simulink subsystem "ElectricalThermalSystem"  (R2024a)
settings: Solver=VariableStepAuto  StartTime=0.0  StopTime=10.0  RelTol=1e-3
undefined symbols (not defined in the file): PlantThrEstCmpPwr, PlntDCDCMass, PlntEMCp, PlntThrAirBpt, PlntThrAirCond, PlntThrAirCp, PlntThrAirCpBpt, PlntThrAirPrand, PlntThrAirRho, PlntThrAirVisc, PlntThrBattDCFlwRatio, PlntThrBattJacArea, PlntThrBattJacLen, PlntThrChArea, PlntThrChDia, PlntThrConvCoeff, PlntThrCoolCond, PlntThrCoolCp, PlntThrCoolCpBpt, PlntThrCoolPrand, PlntThrCoolRho, PlntThrCoolVisc, PlntThrDCJacArea, PlntThrDCJacLen, PlntThrEMJacArea, PlntThrEMJacLen, PlntThrEstCOPLut, PlntThrEstDTLut, PlntThrFanDisp, PlntThrFanMaxSpd, PlntThrFanMechEff, PlntThrFanNomP, PlntThrFanVolEff, PlntThrHeaterMaxPwr, PlntThrHtVsCurr, PlntThrHtVsCurrBpt, PlntThrPmpDisp, PlntThrPmpHeadP, PlntThrPmpMaxSpd, PlntThrPmpMechEff, PlntThrPmpVolEff, PlntThrRadAirArea, PlntThrRadAirDh, PlntThrRadFanAreaFlw, PlntThrRadFlwCoef, PlntThrRadGapHeight, PlntThrRadLength, PlntThrRadNTubes, PlntThrRadTubeDh, PlntThrRadTubeHeight, PlntThrRadWidth
libraries: simulink x5, autolibsharedcommon x1, autolibutils x1
settings Model: ModifiedByFormat=The MathWorks, Inc.  Creator=The MathWorks, Inc.  LastModifiedBy=The MathWorks, Inc.
settings RTWCC: GPUComputeCapability=3.5  LargeConstantGeneration=WriteOnlyDNNConstantsToDataFiles

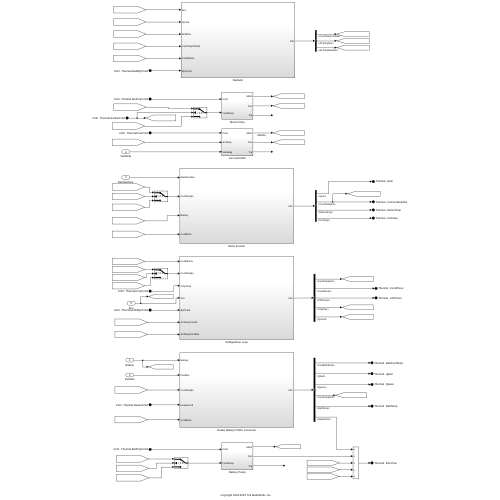
[thumbnail: Simulink's stored preview of the top-level diagram]
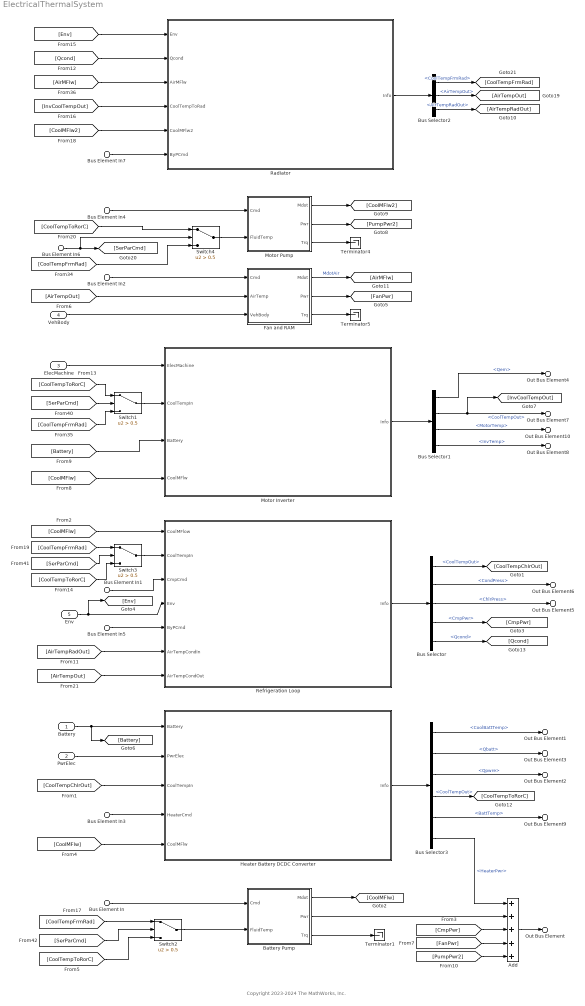
== system ElectricalThermalSystem ==
  note: Copyright 2023-2024 The MathWorks, Inc.
  Battery : Inport
  PwrElec : Inport  Port=2
  ElecMachine : Inport  Port=3
  VehBody : Inport  Port=4
  Env : Inport  Port=5
  Bus Element In : Inport  Port=6  PortName=Cntrl  Element=Thermal.BattPmpCmd
  Bus Element In1 : Inport  Port=6  PortName=Cntrl  Element=Thermal.CmpCmd
  Bus Element In2 : Inport  Port=6  PortName=Cntrl  Element=Thermal.FanCmd
  Bus Element In3 : Inport  Port=6  PortName=Cntrl  Element=Thermal.HeaterCmd
  Bus Element In4 : Inport  Port=6  PortName=Cntrl  Element=Thermal.MotPmpCmd
  Bus Element In5 : Inport  Port=6  PortName=Cntrl  Element=Thermal.ChlrByPCmd
  Bus Element In6 : Inport  Port=6  PortName=Cntrl  Element=Thermal.SerParCmd
  Bus Element In7 : Inport  Port=6  PortName=Cntrl  Element=Thermal.RadByPCmd
  Add : Sum  Inputs=+++++
  Battery Pump : Subsystem
  Bus Selector : BusSelector  OutputSignals=CoolTempOut,CondPress,ChlrPress,CmpPwr,Qcond
  Bus Selector1 : BusSelector  OutputSignals=Qem,CoolTempOut,MotorTemp,InvTemp
  Bus Selector2 : BusSelector  OutputSignals=CoolTempFrmRad,AirTempOut,AirTempRadOut
  Bus Selector3 : BusSelector  OutputSignals=CoolBattTemp,Qbatt,Qpwre,CoolTempOut,BattTemp,HeaterPwr
  Fan and RAM : Subsystem
  Heater Battery DCDC Converter : Subsystem
  Motor Inverter : Subsystem
  Motor Pump : Subsystem
  Radiator : Subsystem
  Refrigeration Loop : Subsystem
  Switch{1..4} (4 alike) : Switch  Criteria=u2 > Threshold  Threshold=0.5  SaturateOnIntegerOverflow=off  InputSameDT=off
  Terminator1 : Terminator
  Terminator4 : Terminator
  Terminator5 : Terminator
  Out Bus Element7 : Outport  PortName=Thermal  Element=InvCoolTempOut
  Out Bus Element8 : Outport  PortName=Thermal  Element=InvTemp
  Out Bus Element9 : Outport  PortName=Thermal  Element=BattTemp
  Out Bus Element10 : Outport  PortName=Thermal  Element=MotorTemp
  Out Bus Element5 : Outport  PortName=Thermal  Element=ChlrPress
  Out Bus Element6 : Outport  PortName=Thermal  Element=CondPress
  Out Bus Element : Outport  PortName=Thermal  Element=EAccPwr
  Out Bus Element1 : Outport  PortName=Thermal  Element=BattCoolTemp
  Out Bus Element3 : Outport  PortName=Thermal  Element=Qbatt
  Out Bus Element2 : Outport  PortName=Thermal  Element=Qpwre
  Out Bus Element4 : Outport  PortName=Thermal  Element=Qem
  wires:
  [CoolTempFrmRad] -> Switch4/3
  [CoolTempToRorC] -> Switch4/1
  [CoolTempToRorC] -> Switch2/3
  [CoolTempFrmRad] -> Switch2/1
  [CoolTempFrmRad] -> Switch1/3
  [CoolTempToRorC] -> Switch1/1
  [CoolTempToRorC] -> Switch3/3
  [CoolTempFrmRad] -> Switch3/1
  Bus Selector3/6 -> Add/1  "<HeaterPwr>"
  Battery Pump/2(Pwr) -> Add/2
  [CmpPwr] -> Add/3
  [FanPwr] -> Add/4
  [PumpPwr2] -> Add/5
  Bus Selector1/4 -> Out Bus Element8/1  "<InvTemp>"
  Bus Selector3/5 -> Out Bus Element9/1  "<BattTemp>"
  Bus Selector1/3 -> Out Bus Element10/1  "<MotorTemp>"
  Bus Selector/1 -> [CoolTempChlrOut]  "<CoolTempOut>"
  Bus Selector2/1 -> [CoolTempFrmRad]  "<CoolTempFrmRad>"
  [CoolMFlw2] -> Radiator/5(CoolMFlw2)
  Switch4/1 -> Motor Pump/2(FluidTemp)
  Bus Element In6/1 -> Switch4/2, [SerParCmd]
  Switch3/1 -> Refrigeration Loop/2(CoolTempIn)
  [SerParCmd] -> Switch3/2
  Switch2/1 -> Battery Pump/2(FluidTemp)
  [SerParCmd] -> Switch2/2
  [SerParCmd] -> Switch1/2
  Switch1/1 -> Motor Inverter/2(CoolTempIn)
  Bus Selector2/2 -> [AirTempOut]  "<AirTempOut>"
  Radiator/1(Info) -> Bus Selector2/1
  [InvCoolTempOut] -> Radiator/4(CoolTempToRad)
  [AirMFlw] -> Radiator/3(AirMFlw)
  [Qcond] -> Radiator/2(Qcond)
  [Env] -> Radiator/1(Env)
  Refrigeration Loop/1(Info) -> Bus Selector/1
  Bus Selector/5 -> [Qcond]  "<Qcond>"
  Motor Pump/1(Mdot) -> [CoolMFlw2]
  Motor Pump/2(Pwr) -> [PumpPwr2]
  Motor Pump/3(Trq) -> Terminator4/1
  Bus Element In4/1 -> Motor Pump/1(Cmd)
  Bus Selector1/2 -> Out Bus Element7/1, [InvCoolTempOut]  "<CoolTempOut>"
  Bus Selector1/1 -> Out Bus Element4/1  "<Qem>"
  Motor Inverter/1(Info) -> Bus Selector1/1
  [Battery] -> Motor Inverter/3(Battery)
  [CoolMFlw] -> Motor Inverter/4(CoolMFlw)
  VehBody/1 -> Fan and RAM/3(VehBody)
  Fan and RAM/3(Trq) -> Terminator5/1
  Fan and RAM/2(Pwr) -> [FanPwr]
  Fan and RAM/1(Mdot) -> [AirMFlw]  "MdotAir"
  Bus Element In2/1 -> Fan and RAM/1(Cmd)
  [AirTempOut] -> Fan and RAM/2(AirTemp)
  [CoolMFlw] -> Heater Battery DCDC Converter/5(CoolMFlw)
  Add/1 -> Out Bus Element/1
  Bus Selector/3 -> Out Bus Element5/1  "<ChlrPress>"
  Bus Selector/2 -> Out Bus Element6/1  "<CondPress>"
  Bus Selector/4 -> [CmpPwr]  "<CmpPwr>"
  [CoolTempChlrOut] -> Heater Battery DCDC Converter/3(CoolTempIn)
  Env/1 -> Refrigeration Loop/4(Env), [Env]
  Bus Element In1/1 -> Refrigeration Loop/3(CmpCmd)
  [CoolMFlw] -> Refrigeration Loop/1(CoolMFlow)
  Bus Selector3/4 -> [CoolTempToRorC]  "<CoolTempOut>"
  Bus Selector3/3 -> Out Bus Element2/1  "<Qpwre>"
  Bus Selector3/2 -> Out Bus Element3/1  "<Qbatt>"
  Bus Selector3/1 -> Out Bus Element1/1  "<CoolBattTemp>"
  Heater Battery DCDC Converter/1(Info) -> Bus Selector3/1
  Bus Element In3/1 -> Heater Battery DCDC Converter/4(HeaterCmd)
  Battery Pump/3(Trq) -> Terminator1/1
  Battery Pump/1(Mdot) -> [CoolMFlw]
  Bus Element In/1 -> Battery Pump/1(Cmd)
  ElecMachine/1 -> Motor Inverter/1(ElecMachine)
  PwrElec/1 -> Heater Battery DCDC Converter/2(PwrElec)
  Battery/1 -> [Battery], Heater Battery DCDC Converter/1(Battery)
  Bus Element In7/1 -> Radiator/6(ByPCmd)
  Bus Element In5/1 -> Refrigeration Loop/5(ByPCmd)
  Bus Selector2/3 -> [AirTempRadOut]  "<AirTempRadOut>"
  [AirTempRadOut] -> Refrigeration Loop/6(AirTempCondIn)
  [AirTempOut] -> Refrigeration Loop/7(AirTempCondOut)

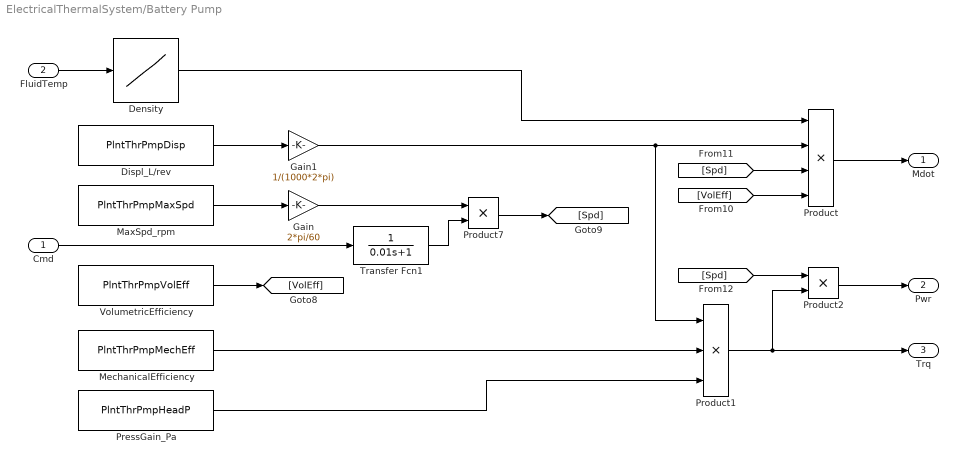
== system ElectricalThermalSystem/Battery Pump ==
  Cmd : Inport
  FluidTemp : Inport  Port=2
  Density : Lookup_n-D  NumberOfTableDimensions=1  BreakpointsForDimension1=PlntThrCoolCpBpt  Table=PlntThrCoolRho  ExtrapMethod=Clip  UseLastTableValue=on  InternalRulePriority=Speed  RndMeth=Simplest
  Displ_L/rev : Constant  Value=PlntThrPmpDisp  SampleTime=-1
  Gain : Gain  Gain=2*pi/60
  Gain1 : Gain  Gain=1/(1000*2*pi)
  MaxSpd_rpm : Constant  Value=PlntThrPmpMaxSpd  SampleTime=-1
  MechanicalEfficiency : Constant  Value=PlntThrPmpMechEff  SampleTime=-1
  PressGain_Pa : Constant  Value=PlntThrPmpHeadP  SampleTime=-1
  Product : Product  Inputs=4
  Product1 : Product  Inputs=3
  Product2 : Product
  Product7 : Product
  Transfer Fcn1 : TransferFcn  Denominator=[0.01 1]
  VolumetricEfficiency : Constant  Value=PlntThrPmpVolEff  SampleTime=-1
  Mdot : Outport
  Pwr : Outport  Port=2
  Trq : Outport  Port=3
  wires:
  Product2/1 -> Pwr/1
  Cmd/1 -> Transfer Fcn1/1
  Product/1 -> Mdot/1
  Gain1/1 -> Product/2, Product1/1
  Product1/1 -> Product2/2, Trq/1
  PressGain_Pa/1 -> Product1/3
  [Spd] -> Product2/1
  MechanicalEfficiency/1 -> Product1/2
  [VolEff] -> Product/4
  [Spd] -> Product/3
  Product7/1 -> [Spd]
  Displ_L/rev/1 -> Gain1/1
  Gain/1 -> Product7/1
  MaxSpd_rpm/1 -> Gain/1
  Density/1 -> Product/1
  VolumetricEfficiency/1 -> [VolEff]
  FluidTemp/1 -> Density/1
  Transfer Fcn1/1 -> Product7/2

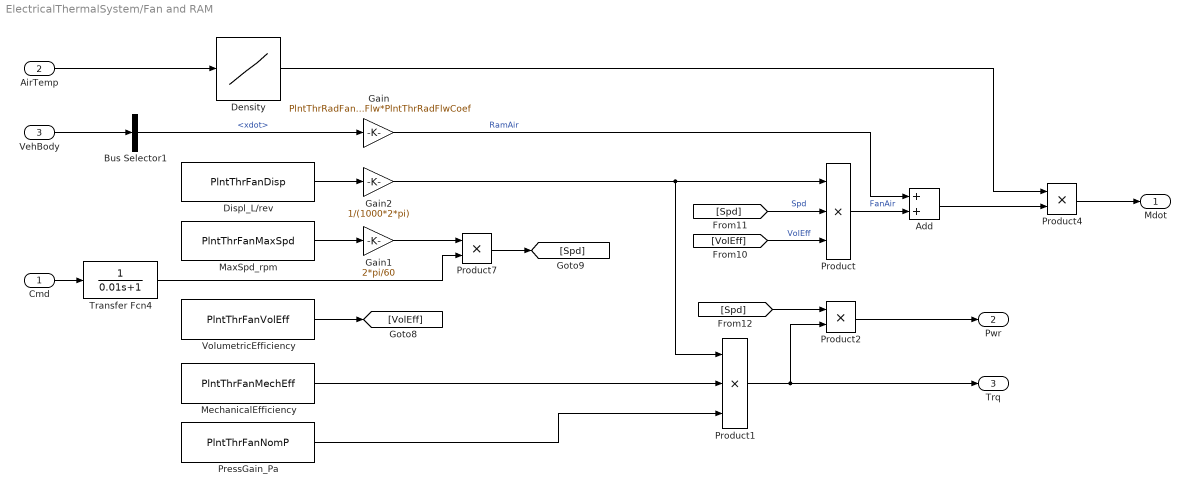
== system ElectricalThermalSystem/Fan and RAM ==
  Cmd : Inport
  AirTemp : Inport  Port=2
  VehBody : Inport  Port=3
  Add : Sum
  Bus Selector1 : BusSelector  OutputSignals=BdyFrm.Cg.Vel.xdot
  Density : Lookup_n-D  NumberOfTableDimensions=1  BreakpointsForDimension1=PlntThrAirBpt  Table=PlntThrAirRho  ExtrapMethod=Clip  UseLastTableValue=on  InternalRulePriority=Speed  RndMeth=Simplest
  Displ_L/rev : Constant  Value=PlntThrFanDisp  SampleTime=-1
  Gain : Gain  Gain=PlntThrRadFanAreaFlw*PlntThrRadFlwCoef
  Gain1 : Gain  Gain=2*pi/60
  Gain2 : Gain  Gain=1/(1000*2*pi)
  MaxSpd_rpm : Constant  Value=PlntThrFanMaxSpd  SampleTime=-1
  MechanicalEfficiency : Constant  Value=PlntThrFanMechEff  SampleTime=-1
  PressGain_Pa : Constant  Value=PlntThrFanNomP  SampleTime=-1
  Product : Product  Inputs=3
  Product1 : Product  Inputs=3
  Product2 : Product
  Product4 : Product
  Product7 : Product
  Transfer Fcn4 : TransferFcn  Denominator=[0.01 1]
  VolumetricEfficiency : Constant  Value=PlntThrFanVolEff  SampleTime=-1
  Mdot : Outport
  Pwr : Outport  Port=2
  Trq : Outport  Port=3
  wires:
  Gain/1 -> Add/1  "RamAir"
  Add/1 -> Product4/2
  Product4/1 -> Mdot/1
  [Spd] -> Product/2  "Spd"
  [VolEff] -> Product/3  "VolEff"
  Product2/1 -> Pwr/1
  Cmd/1 -> Transfer Fcn4/1
  Gain2/1 -> Product/1, Product1/1
  Product1/1 -> Product2/2, Trq/1
  PressGain_Pa/1 -> Product1/3
  [Spd] -> Product2/1
  MechanicalEfficiency/1 -> Product1/2
  Product7/1 -> [Spd]
  Displ_L/rev/1 -> Gain2/1
  Gain1/1 -> Product7/1
  MaxSpd_rpm/1 -> Gain1/1
  Density/1 -> Product4/1
  VolumetricEfficiency/1 -> [VolEff]
  VehBody/1 -> Bus Selector1/1
  Bus Selector1/1 -> Gain/1  "<xdot>"
  Product/1 -> Add/2  "FanAir"
  AirTemp/1 -> Density/1
  Transfer Fcn4/1 -> Product7/2

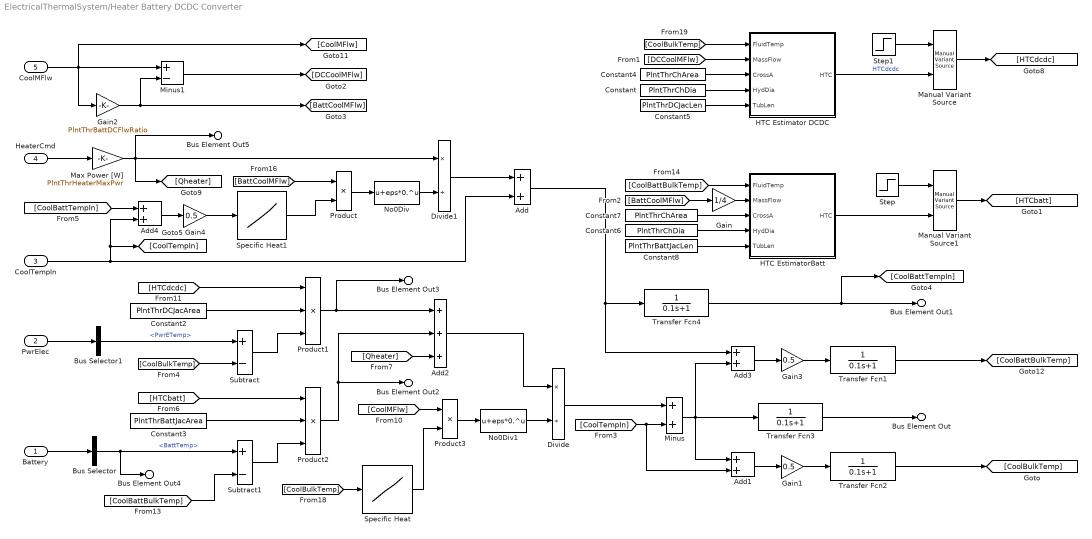
== system ElectricalThermalSystem/Heater Battery DCDC Converter ==
  Battery : Inport
  PwrElec : Inport  Port=2
  CoolTempIn : Inport  Port=3
  HeaterCmd : Inport  Port=4
  CoolMFlw : Inport  Port=5
  Add{,1,3..4} (4 alike) : Sum
  Add2 : Sum  Inputs=+++
  Bus Selector : BusSelector  OutputSignals=BattInfo.BattTemp
  Bus Selector1 : BusSelector  OutputSignals=PwrETemp
  Constant : Constant  Value=PlntThrChDia  SampleTime=-1
  Constant2 : Constant  Value=PlntThrDCJacArea  SampleTime=-1
  Constant3 : Constant  Value=PlntThrBattJacArea  SampleTime=-1
  Constant4 : Constant  Value=PlntThrChArea  SampleTime=-1
  Constant5 : Constant  Value=PlntThrDCJacLen  SampleTime=-1
  Constant6 : Constant  Value=PlntThrChDia  SampleTime=-1
  Constant7 : Constant  Value=PlntThrChArea  SampleTime=-1
  Constant8 : Constant  Value=PlntThrBattJacLen  SampleTime=-1
  Divide : Product  Inputs=*/
  Divide1 : Product  Inputs=*/
  Gain : Gain  Gain=1/4
  Gain1 : Gain  Gain=0.5
  Gain2 : Gain  Gain=PlntThrBattDCFlwRatio
  Gain3 : Gain  Gain=0.5
  Gain4 : Gain  Gain=0.5
  HTC Estimator DCDC : Subsystem
  HTC EstimatorBatt : Subsystem
  Manual Variant Source : simulink/Signal Routing/Manual Variant Source  NumChoices=2  LabelModeActiveChoice=V_2
  Manual Variant Source1 : simulink/Signal Routing/Manual Variant Source  NumChoices=2  LabelModeActiveChoice=V_2
  Max Power [W] : Gain  Gain=PlntThrHeaterMaxPwr
  Minus : Sum
  Minus1 : Sum  Inputs=+-
  No0Div : Fcn  Expr=u+eps*0.^u
  No0Div1 : Fcn  Expr=u+eps*0.^u
  Product : Product
  Product1 : Product  Inputs=3
  Product2 : Product  Inputs=3
  Product3 : Product
  Specific Heat : Lookup_n-D  NumberOfTableDimensions=1  BreakpointsForDimension1=PlntThrCoolCpBpt  Table=PlntThrCoolCp  ExtrapMethod=Clip  UseLastTableValue=on  InternalRulePriority=Speed  RndMeth=Simplest
  Specific Heat1 : Lookup_n-D  NumberOfTableDimensions=1  BreakpointsForDimension1=PlntThrCoolCpBpt  Table=PlntThrCoolCp  ExtrapMethod=Clip  UseLastTableValue=on  InternalRulePriority=Speed  RndMeth=Simplest
  Step : Step  Time=0.1  After=PlntThrConvCoeff*0+2100  SampleTime=0
  Step1 : Step  Time=0.1  After=PlntThrConvCoeff*2  SampleTime=0
  Subtract : Sum  Inputs=+-
  Subtract1 : Sum  Inputs=+-
  Transfer Fcn{1..4} (4 alike) : TransferFcn  Denominator=[0.1 1]
  Bus Element Out : Outport  PortName=Info  Element=CoolTempOut
  Bus Element Out1 : Outport  PortName=Info  Element=CoolBattTemp
  Bus Element Out2 : Outport  PortName=Info  Element=Qbatt
  Bus Element Out3 : Outport  PortName=Info  Element=Qpwre
  Bus Element Out4 : Outport  PortName=Info  Element=BattTemp
  Bus Element Out5 : Outport  PortName=Info  Element=HeaterPwr
  wires:
  Step/1 -> Manual Variant Source1/1
  HeaterCmd/1 -> Max Power [W]/1
  Battery/1 -> Bus Selector/1
  PwrElec/1 -> Bus Selector1/1
  Max Power [W]/1 -> [Qheater], Divide1/1, Bus Element Out5/1
  Manual Variant Source/1 -> [HTCdcdc]
  HTC Estimator DCDC/1(HTC) -> Manual Variant Source/2  "HTCdcdc"
  HTC EstimatorBatt/1(HTC) -> Manual Variant Source1/2
  Manual Variant Source1/1 -> [HTCbatt]
  Gain2/1 -> Minus1/2, [BattCoolMFlw]
  [CoolBulkTemp] -> Subtract/2
  [HTCdcdc] -> Product1/1
  Constant2/1 -> Product1/2
  Subtract/1 -> Product1/3
  Constant3/1 -> Product2/2
  Subtract1/1 -> Product2/3
  Product1/1 -> Bus Element Out3/1, Add2/1
  Product2/1 -> Bus Element Out2/1, Add2/2
  Add2/1 -> Divide/1
  Divide/1 -> Minus/1
  [CoolTempIn] -> Add1/2, Minus/2
  Minus/1 -> Transfer Fcn3/1, Add1/1, Add3/2
  Add3/1 -> Gain3/1
  [CoolBattBulkTemp] -> Subtract1/2
  CoolMFlw/1 -> [CoolMFlw], Minus1/1, Gain2/1
  Minus1/1 -> [DCCoolMFlw]
  CoolTempIn/1 -> Add/2, Add4/2, [CoolTempIn]
  Divide1/1 -> Add/1
  Add/1 -> Add3/1, Transfer Fcn4/1
  [Qheater] -> Add2/3
  Add1/1 -> Gain1/1
  [CoolBulkTemp] -> Specific Heat/1
  Bus Selector1/1 -> Subtract/1  "<PwrETemp>"
  Bus Selector/1 -> Bus Element Out4/1, Subtract1/1  "<BattTemp>"
  Gain3/1 -> Transfer Fcn1/1
  Transfer Fcn1/1 -> [CoolBattBulkTemp]
  Gain1/1 -> Transfer Fcn2/1
  Transfer Fcn2/1 -> [CoolBulkTemp]
  Transfer Fcn3/1 -> Bus Element Out/1
  Product/1 -> No0Div/1
  [BattCoolMFlw] -> Product/1
  Specific Heat1/1 -> Product/2
  No0Div/1 -> Divide1/2
  Product3/1 -> No0Div1/1
  No0Div1/1 -> Divide/2
  [CoolMFlw] -> Product3/1
  Specific Heat/1 -> Product3/2
  [HTCbatt] -> Product2/1
  Add4/1 -> Gain4/1
  Gain4/1 -> Specific Heat1/1
  Transfer Fcn4/1 -> [CoolBattTempIn], Bus Element Out1/1
  [CoolBattTempIn] -> Add4/1
  Step1/1 -> Manual Variant Source/1
  [CoolBulkTemp] -> HTC Estimator DCDC/1(FluidTemp)
  [DCCoolMFlw] -> HTC Estimator DCDC/2(MassFlow)
  Constant/1 -> HTC Estimator DCDC/4(HydDia)
  Constant4/1 -> HTC Estimator DCDC/3(CrossA)
  Constant5/1 -> HTC Estimator DCDC/5(TubLen)
  Constant7/1 -> HTC EstimatorBatt/3(CrossA)
  Constant6/1 -> HTC EstimatorBatt/4(HydDia)
  Constant8/1 -> HTC EstimatorBatt/5(TubLen)
  Gain/1 -> HTC EstimatorBatt/2(MassFlow)
  [BattCoolMFlw] -> Gain/1
  [CoolBattBulkTemp] -> HTC EstimatorBatt/1(FluidTemp)

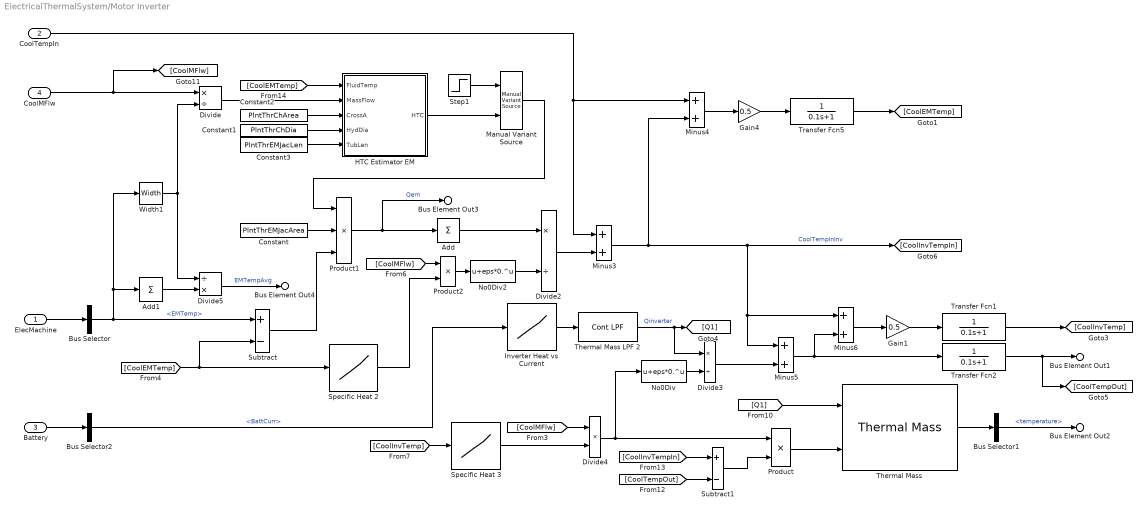
== system ElectricalThermalSystem/Motor Inverter ==
  ElecMachine : Inport
  CoolTempIn : Inport  Port=2
  Battery : Inport  Port=3
  CoolMFlw : Inport  Port=4
  Add : Sum  Inputs=1
  Add1 : Sum  Inputs=1
  Bus Selector : BusSelector  OutputSignals=EMTemp
  Bus Selector1 : BusSelector  OutputSignals=temperature
  Bus Selector2 : BusSelector  OutputSignals=BattInfo.BattCurr
  Constant : Constant  Value=PlntThrEMJacArea  SampleTime=-1
  Constant1 : Constant  Value=PlntThrChDia
  Constant2 : Constant  Value=PlntThrChArea
  Constant3 : Constant  Value=PlntThrEMJacLen
  Divide : Product  Inputs=*/
  Divide2 : Product  Inputs=*/
  Divide3 : Product  Inputs=*/
  Divide4 : Product
  Divide5 : Product  Inputs=/*
  Gain1 : Gain  Gain=0.5
  Gain4 : Gain  Gain=0.5
  HTC Estimator EM : Subsystem
  Inverter Heat vs Current : Lookup_n-D  NumberOfTableDimensions=1  BreakpointsForDimension1=PlntThrHtVsCurrBpt  IndexSearchMethod=Linear search  BeginIndexSearchUsingPreviousIndexResult=on  Table=PlntThrHtVsCurr  ExtrapMethod=Clip  UseLastTableValue=on  InternalRulePriority=Speed  RndMeth=Simplest
  Manual Variant Source : simulink/Signal Routing/Manual Variant Source  NumChoices=2  LabelModeActiveChoice=V_2
  Minus{3..6} (4 alike) : Sum
  No0Div : Fcn  Expr=u+eps*0.^u
  No0Div2 : Fcn  Expr=u+eps*0.^u
  Product : Product
  Product1 : Product  Inputs=3
  Product2 : Product
  Specific Heat 2 : Lookup_n-D  NumberOfTableDimensions=1  BreakpointsForDimension1=PlntThrCoolCpBpt  Table=PlntThrCoolCp  ExtrapMethod=Clip  UseLastTableValue=on  InternalRulePriority=Speed  RndMeth=Simplest
  Specific Heat 3 : Lookup_n-D  NumberOfTableDimensions=1  BreakpointsForDimension1=PlntThrCoolCpBpt  Table=PlntThrCoolCp  ExtrapMethod=Clip  UseLastTableValue=on  InternalRulePriority=Speed  RndMeth=Simplest
  Step1 : Step  Time=0.1  After=PlntThrConvCoeff  SampleTime=0
  Subtract : Sum  Inputs=+-
  Subtract1 : Sum  Inputs=+-
  Thermal Mass : autolibsharedcommon/Thermal Mass  MassOrVol=Mass  Mass=2*PlntDCDCMass  Volume=0.01  Rho=997  HeatCp=PlntEMCp*ones(1,2)  HeatBrkPts=PlntBattCpBpt  Tinit=EnvAirTemp  Tenv=EnvAirTemp  ConvHTC=1  EnvArea=0.1
  Thermal Mass LPF 2 : autolibutils/Cont LPF  wc=2  AbsoluteTolerance=auto  aMode=6
  Transfer Fcn1 : TransferFcn  Denominator=[0.1 1]
  Transfer Fcn2 : TransferFcn  Denominator=[0.1 1]
  Transfer Fcn5 : TransferFcn  Denominator=[0.1 1]
  Width1 : Width
  Bus Element Out3 : Outport  PortName=Info  Element=Qem
  Bus Element Out1 : Outport  PortName=Info  Element=CoolTempOut
  Bus Element Out4 : Outport  PortName=Info  Element=MotorTemp
  Bus Element Out2 : Outport  PortName=Info  Element=InvTemp
  wires:
  ElecMachine/1 -> Bus Selector/1
  Step1/1 -> Manual Variant Source/1
  HTC Estimator EM/1(HTC) -> Manual Variant Source/2
  Manual Variant Source/1 -> Product1/1
  [CoolEMTemp] -> HTC Estimator EM/1(FluidTemp)
  CoolMFlw/1 -> [CoolMFlw], Divide/1
  Constant1/1 -> HTC Estimator EM/4(HydDia)
  Subtract/1 -> Product1/3
  Product1/1 -> Bus Element Out3/1, Add/1  "Qem"
  Bus Selector/1 -> Width1/1, Add1/1, Subtract/1  "<EMTemp>"
  Battery/1 -> Bus Selector2/1
  Bus Selector2/1 -> Inverter Heat vs Current/1  "<BattCurr>"
  Add/1 -> Divide2/1
  Divide2/1 -> Minus3/2
  Minus4/1 -> Gain4/1
  Minus3/1 -> Minus6/1, Minus5/1, [CoolInvTempIn], Minus4/2  "CoolTempInInv"
  CoolTempIn/1 -> Minus4/1, Minus3/1
  [CoolEMTemp] -> Specific Heat 2/1, Subtract/2
  Inverter Heat vs Current/1 -> Thermal Mass LPF 2/1
  Divide3/1 -> Minus5/2
  Minus6/1 -> Gain1/1
  Minus5/1 -> Transfer Fcn2/1, Minus6/2
  [CoolInvTemp] -> Specific Heat 3/1
  Width1/1 -> Divide/2, Divide5/1
  Divide/1 -> HTC Estimator EM/2(MassFlow)
  Add1/1 -> Divide5/2
  Divide5/1 -> Bus Element Out4/1  "EMTempAvg"
  Specific Heat 3/1 -> Divide4/2
  [CoolMFlw] -> Divide4/1
  Divide4/1 -> Product/1, No0Div/1
  [CoolInvTempIn] -> Subtract1/1
  [CoolTempOut] -> Subtract1/2
  Subtract1/1 -> Product/2
  Thermal Mass/1 -> Bus Selector1/1
  Transfer Fcn5/1 -> [CoolEMTemp]
  Gain4/1 -> Transfer Fcn5/1
  Transfer Fcn2/1 -> [CoolTempOut], Bus Element Out1/1
  Transfer Fcn1/1 -> [CoolInvTemp]
  Gain1/1 -> Transfer Fcn1/1
  [Q1] -> Thermal Mass/1
  Bus Selector1/1 -> Bus Element Out2/1  "<temperature>"
  No0Div/1 -> Divide3/2
  Product2/1 -> No0Div2/1
  No0Div2/1 -> Divide2/2
  [CoolMFlw] -> Product2/1
  Specific Heat 2/1 -> Product2/2
  Product/1 -> Thermal Mass/2
  Thermal Mass LPF 2/1 -> [Q1], Divide3/1  "Qinverter"
  Constant/1 -> Product1/2
  Constant2/1 -> HTC Estimator EM/3(CrossA)
  Constant3/1 -> HTC Estimator EM/5(TubLen)

== system ElectricalThermalSystem/Motor Pump ==
  Cmd : Inport
  FluidTemp : Inport  Port=2
  Density : Lookup_n-D  NumberOfTableDimensions=1  BreakpointsForDimension1=PlntThrCoolCpBpt  Table=PlntThrCoolRho  ExtrapMethod=Clip  UseLastTableValue=on  InternalRulePriority=Speed  RndMeth=Simplest
  Displ_L/rev : Constant  Value=PlntThrPmpDisp  SampleTime=-1
  Gain : Gain  Gain=2*pi/60
  Gain1 : Gain  Gain=1/(1000*2*pi)
  MaxSpd_rpm : Constant  Value=PlntThrPmpMaxSpd  SampleTime=-1
  MechanicalEfficiency : Constant  Value=PlntThrPmpMechEff  SampleTime=-1
  PressGain_Pa : Constant  Value=PlntThrPmpHeadP  SampleTime=-1
  Product : Product  Inputs=4
  Product1 : Product  Inputs=3
  Product2 : Product
  Product7 : Product
  Transfer Fcn2 : TransferFcn  Denominator=[0.01 1]
  VolumetricEfficiency : Constant  Value=PlntThrPmpVolEff  SampleTime=-1
  Mdot : Outport
  Pwr : Outport  Port=2
  Trq : Outport  Port=3
  wires:
  Product2/1 -> Pwr/1
  Cmd/1 -> Transfer Fcn2/1
  Product/1 -> Mdot/1
  Gain1/1 -> Product/2, Product1/1
  Product1/1 -> Product2/2, Trq/1
  PressGain_Pa/1 -> Product1/3
  [Spd] -> Product2/1
  MechanicalEfficiency/1 -> Product1/2
  [VolEff] -> Product/4
  [Spd] -> Product/3
  Product7/1 -> [Spd]
  Displ_L/rev/1 -> Gain1/1
  Gain/1 -> Product7/1
  MaxSpd_rpm/1 -> Gain/1
  Density/1 -> Product/1
  VolumetricEfficiency/1 -> [VolEff]
  FluidTemp/1 -> Density/1
  Transfer Fcn2/1 -> Product7/2

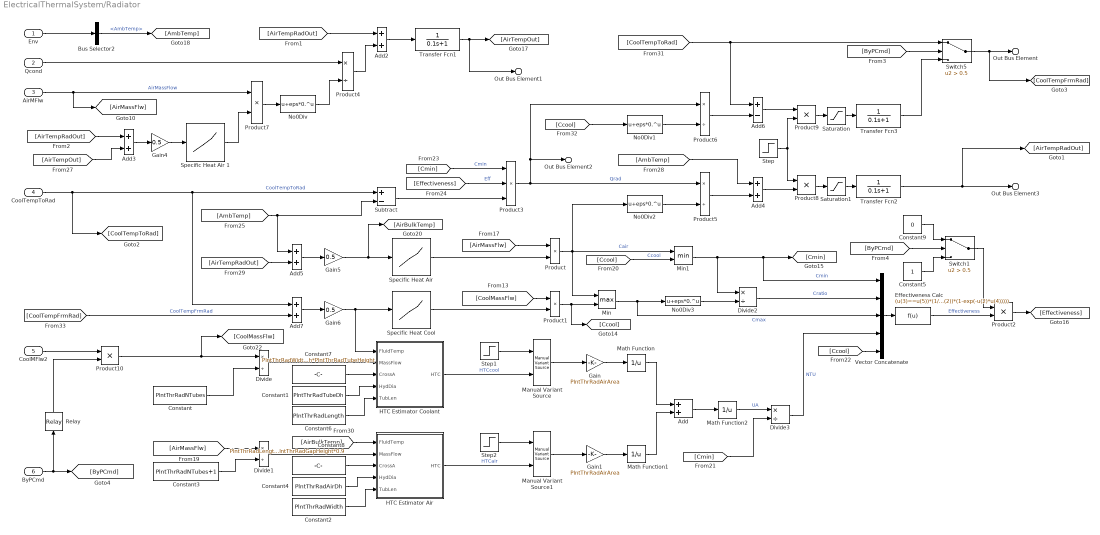
== system ElectricalThermalSystem/Radiator ==
  Env : Inport
  Qcond : Inport  Port=2
  AirMFlw : Inport  Port=3
  CoolTempToRad : Inport  Port=4
  CoolMFlw2 : Inport  Port=5
  ByPCmd : Inport  Port=6
  Add{,2..5,7} (6 alike) : Sum
  Add6 : Sum  Inputs=+-
  Bus Selector2 : BusSelector  OutputSignals=AmbTemp
  Constant : Constant  Value=PlntThrRadNTubes  SampleTime=-1
  Constant1 : Constant  Value=PlntThrRadTubeDh  SampleTime=-1
  Constant2 : Constant  Value=PlntThrRadWidth  SampleTime=-1
  Constant3 : Constant  Value=PlntThrRadNTubes+1  SampleTime=-1
  Constant4 : Constant  Value=PlntThrRadAirDh  SampleTime=-1
  Constant5 : Constant  SampleTime=-1
  Constant6 : Constant  Value=PlntThrRadLength  SampleTime=-1
  Constant7 : Constant  Value=PlntThrRadWidth*PlntThrRadTubeHeight  SampleTime=-1
  Constant8 : Constant  Value=PlntThrRadLength*PlntThrRadGapHeight*0.9  SampleTime=-1
  Constant9 : Constant  Value=0  SampleTime=-1
  Divide : Product  Inputs=*/
  Divide1 : Product  Inputs=*/
  Divide2 : Product  Inputs=*/  RndMeth=Zero  SaturateOnIntegerOverflow=on
  Divide3 : Product  Inputs=*/
  Effectiveness Calc : Fcn  Expr=(u(3)==u(5))*(1/u(2))*(1-exp(-u(2)*(1-exp(-u(4)))))+(u(1)==u(5))*(1-exp((-1/u(2))*(1-exp(-u(2)*u(4)))))
  Gain : Gain  Gain=PlntThrRadAirArea
  Gain1 : Gain  Gain=PlntThrRadAirArea
  Gain4 : Gain  Gain=0.5
  Gain5 : Gain  Gain=0.5
  Gain6 : Gain  Gain=0.5
  HTC Estimator Air : Subsystem
  HTC Estimator Coolant : Subsystem
  Manual Variant Source : simulink/Signal Routing/Manual Variant Source  NumChoices=2  LabelModeActiveChoice=V_2
  Manual Variant Source1 : simulink/Signal Routing/Manual Variant Source  NumChoices=2  LabelModeActiveChoice=V_2
  Math Function : Math  Operator=reciprocal
  Math Function1 : Math  Operator=reciprocal
  Math Function2 : Math  Operator=reciprocal
  Min : MinMax  Function=max  Inputs=2
  Min1 : MinMax  Inputs=2
  No0Div{,1..3} (4 alike) : Fcn  Expr=u+eps*0.^u
  Product{,1..2,7..10} (7 alike) : Product
  Product3 : Product  Inputs=3
  Product4 : Product  Inputs=*/
  Product5 : Product  Inputs=*/
  Product6 : Product  Inputs=*/
  Relay : Relay  OnSwitchValue=0.5  OffSwitchValue=0.5  OnOutputValue=eps  OffOutputValue=1
  Saturation : Saturate  UpperLimit=inf  LowerLimit=173.15
  Saturation1 : Saturate  UpperLimit=inf  LowerLimit=173.15
  Specific Heat Air : Lookup_n-D  NumberOfTableDimensions=1  BreakpointsForDimension1=PlntThrAirCpBpt  Table=PlntThrAirCp  ExtrapMethod=Clip  UseLastTableValue=on  InternalRulePriority=Speed  RndMeth=Simplest
  Specific Heat Air 1 : Lookup_n-D  NumberOfTableDimensions=1  BreakpointsForDimension1=PlntThrAirCpBpt  Table=PlntThrAirCp  ExtrapMethod=Clip  UseLastTableValue=on  InternalRulePriority=Speed  RndMeth=Simplest
  Specific Heat Cool : Lookup_n-D  NumberOfTableDimensions=1  BreakpointsForDimension1=PlntThrCoolCpBpt  Table=PlntThrCoolCp  ExtrapMethod=Clip  UseLastTableValue=on  InternalRulePriority=Speed  RndMeth=Simplest
  Step : Step  SampleTime=0
  Step1 : Step  Time=0.1  After=PlntThrConvCoeff  SampleTime=0
  Step2 : Step  Time=0.1  After=PlntThrConvCoeff  SampleTime=0
  Subtract : Sum  Inputs=+-
  Switch1 : Switch  Criteria=u2 > Threshold  Threshold=0.5  SaturateOnIntegerOverflow=off  InputSameDT=off
  Switch5 : Switch  Criteria=u2 > Threshold  Threshold=0.5  SaturateOnIntegerOverflow=off  InputSameDT=off
  Transfer Fcn1 : TransferFcn  Denominator=[0.1 1]
  Transfer Fcn2 : TransferFcn  Denominator=[0.1 1]
  Transfer Fcn3 : TransferFcn  Denominator=[0.1 1]
  Vector Concatenate : Concatenate  NumInputs=5
  Out Bus Element : Outport  PortName=Info  Element=CoolTempFrmRad
  Out Bus Element1 : Outport  PortName=Info  Element=AirTempOut
  Out Bus Element2 : Outport  PortName=Info  Element=Qrad
  Out Bus Element3 : Outport  PortName=Info  Element=AirTempRadOut
  wires:
  Product2/1 -> [Effectiveness]
  Switch1/1 -> Product2/1
  Constant9/1 -> Switch1/1
  Constant5/1 -> Switch1/3
  [ByPCmd] -> Switch1/2
  [ByPCmd] -> Switch5/2
  ByPCmd/1 -> Relay/1, [ByPCmd]
  Switch5/1 -> Out Bus Element/1, [CoolTempFrmRad]
  Math Function1/1 -> Add/2
  Math Function/1 -> Add/1
  Add/1 -> Math Function2/1
  Product8/1 -> Saturation1/1
  Saturation1/1 -> Transfer Fcn2/1
  Product9/1 -> Saturation/1
  Saturation/1 -> Transfer Fcn3/1
  Add4/1 -> Product8/2
  Add6/1 -> Product9/1
  Step/1 -> Product8/1, Product9/2
  [AirTempRadOut] -> Add2/1
  Gain5/1 -> [AirBulkTemp], Specific Heat Air/1
  Product/1 -> No0Div2/1, Min1/1, Min/1  "Cair"
  Constant2/1 -> HTC Estimator Air/5(TubLen)
  Gain6/1 -> HTC Estimator Coolant/1(FluidTemp), Specific Heat Cool/1
  Vector Concatenate/1 -> Effectiveness Calc/1
  Specific Heat Air/1 -> Product/2
  AirMFlw/1 -> Product7/1, [AirMassFlw]  "AirMassFlow"
  Specific Heat Cool/1 -> Product1/2
  Min/1 -> Vector Concatenate/3, No0Div3/1  "Cmax"
  CoolTempToRad/1 -> Add7/1, Subtract/1, [CoolTempToRad]  "CoolTempToRad"
  [AmbTemp] -> Add4/1
  Min1/1 -> Vector Concatenate/1, [Cmin], Divide2/1  "Cmin"
  Product10/1 -> [CoolMassFlw], Divide/1
  [AmbTemp] -> Add5/1, Subtract/2
  Constant/1 -> Divide/2
  [CoolTempToRad] -> Add6/1, Switch5/1
  Step2/1 -> Manual Variant Source1/1
  Product6/1 -> Add6/2
  [Ccool] -> Min1/2  "Ccool"
  Gain4/1 -> Specific Heat Air 1/1
  Add3/1 -> Gain4/1
  [AirMassFlw] -> Divide1/1
  [AirTempRadOut] -> Add3/1
  Constant4/1 -> HTC Estimator Air/4(HydDia)
  Product1/1 -> [Ccool], Min/2
  Gain/1 -> Math Function/1
  [AirMassFlw] -> Product/1
  Bus Selector2/1 -> [AmbTemp]  "<AmbTemp>"
  HTC Estimator Air/1(HTC) -> Manual Variant Source1/2  "HTCair"
  [AirTempRadOut] -> Add5/2
  HTC Estimator Coolant/1(HTC) -> Manual Variant Source/2  "HTCcool"
  Divide/1 -> HTC Estimator Coolant/2(MassFlow)
  Manual Variant Source/1 -> Gain/1
  [CoolMassFlw] -> Product1/1
  Constant3/1 -> Divide1/2
  Divide1/1 -> HTC Estimator Air/2(MassFlow)
  Step1/1 -> Manual Variant Source/1
  [Ccool] -> No0Div1/1
  Subtract/1 -> Product3/3
  Gain1/1 -> Math Function1/1
  Manual Variant Source1/1 -> Gain1/1
  Add5/1 -> Gain5/1
  Divide2/1 -> Vector Concatenate/2  "Cratio"
  [Ccool] -> Vector Concatenate/5
  [Cmin] -> Divide3/2
  Effectiveness Calc/1 -> Product2/2  "Effectiveness"
  [Cmin] -> Product3/1  "Cmin"
  Product5/1 -> Add4/2
  [AirBulkTemp] -> HTC Estimator Air/1(FluidTemp)
  Product4/1 -> Add2/2
  [AirTempOut] -> Add3/2
  Add7/1 -> Gain6/1
  Env/1 -> Bus Selector2/1
  Qcond/1 -> Product4/1
  Transfer Fcn2/1 -> [AirTempRadOut], Out Bus Element3/1
  Add2/1 -> Transfer Fcn1/1
  Transfer Fcn1/1 -> Out Bus Element1/1, [AirTempOut]
  Specific Heat Air 1/1 -> Product7/2
  Product7/1 -> No0Div/1
  No0Div/1 -> Product4/2
  No0Div1/1 -> Product6/2
  No0Div2/1 -> Product5/2
  No0Div3/1 -> Divide2/2
  [CoolTempFrmRad] -> Add7/2  "CoolTempFrmRad"
  Transfer Fcn3/1 -> Switch5/3
  Product3/1 -> Out Bus Element2/1, Product6/1, Product5/1  "Qrad"
  [Effectiveness] -> Product3/2  "Eff"
  Constant1/1 -> HTC Estimator Coolant/4(HydDia)
  Constant6/1 -> HTC Estimator Coolant/5(TubLen)
  Constant7/1 -> HTC Estimator Coolant/3(CrossA)
  Constant8/1 -> HTC Estimator Air/3(CrossA)
  Math Function2/1 -> Divide3/1  "UA"
  Divide3/1 -> Vector Concatenate/4  "NTU"
  CoolMFlw2/1 -> Product10/1
  Relay/1 -> Product10/2

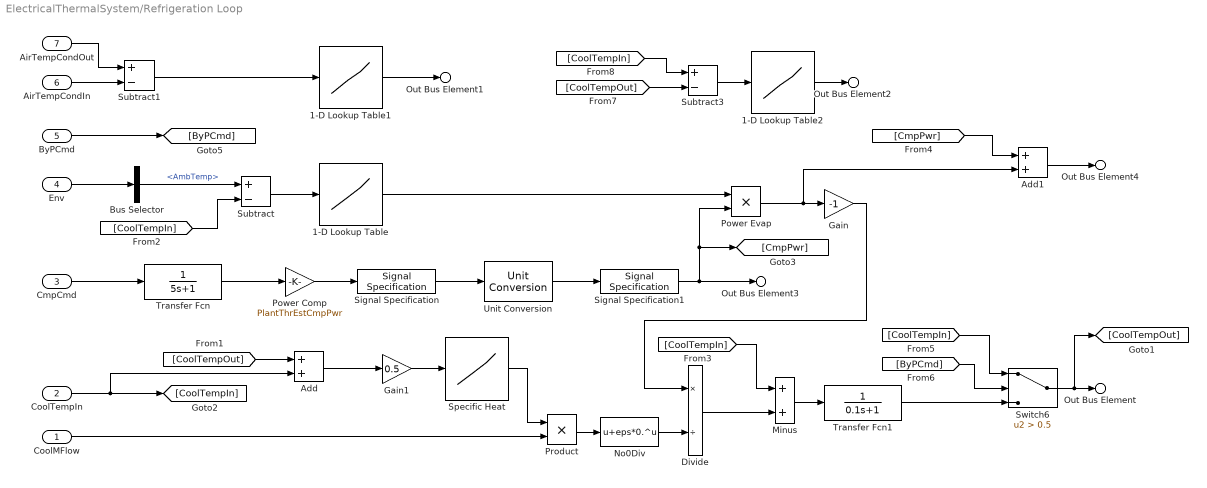
== system ElectricalThermalSystem/Refrigeration Loop ==
  CoolMFlow : Inport
  CoolTempIn : Inport  Port=2
  CmpCmd : Inport  Port=3
  Env : Inport  Port=4
  ByPCmd : Inport  Port=5
  AirTempCondIn : Inport  Port=6
  AirTempCondOut : Inport  Port=7
  1-D Lookup Table : Lookup_n-D  NumberOfTableDimensions=1  BreakpointsForDimension1=PlntThrEstDTLut  Table=PlntThrEstCOPLut  ExtrapMethod=Clip  InternalRulePriority=Speed  RndMeth=Simplest
  1-D Lookup Table1 : Lookup_n-D  NumberOfTableDimensions=1  BreakpointsForDimension1=[0 4.5 10 13 20]  Table=[1.3 1.3 1.53 1.62 1.7]  ExtrapMethod=Clip  UseLastTableValue=on  InternalRulePriority=Speed  RndMeth=Simplest
  1-D Lookup Table2 : Lookup_n-D  NumberOfTableDimensions=1  BreakpointsForDimension1=[0 1 3 7]  Table=[0.65 0.45 0.3 0.3]  ExtrapMethod=Clip  UseLastTableValue=on  InternalRulePriority=Speed  RndMeth=Simplest
  Add : Sum
  Add1 : Sum
  Bus Selector : BusSelector  OutputSignals=AmbTemp
  Divide : Product  Inputs=*/
  Gain : Gain  Gain=-1
  Gain1 : Gain  Gain=0.5
  Minus : Sum
  No0Div : Fcn  Expr=u+eps*0.^u
  Power Comp : Gain  Gain=PlantThrEstCmpPwr
  Power Evap : Product
  Product : Product
  Signal Specification : SignalSpecification  Unit=kW
  Signal Specification1 : SignalSpecification  Unit=watt
  Specific Heat : Lookup_n-D  NumberOfTableDimensions=1  BreakpointsForDimension1=PlntThrCoolCpBpt  Table=PlntThrCoolCp  ExtrapMethod=Clip  UseLastTableValue=on  InternalRulePriority=Speed  RndMeth=Simplest
  Subtract : Sum  Inputs=+-
  Subtract1 : Sum  Inputs=+-
  Subtract3 : Sum  Inputs=+-
  Switch6 : Switch  Criteria=u2 > Threshold  Threshold=0.5  SaturateOnIntegerOverflow=off  InputSameDT=off
  Transfer Fcn : TransferFcn  Denominator=[5 1]
  Transfer Fcn1 : TransferFcn  Denominator=[0.1 1]
  Unit Conversion : UnitConversion
  Out Bus Element : Outport  PortName=Info  Element=CoolTempOut
  Out Bus Element1 : Outport  PortName=Info  Element=CondPress
  Out Bus Element2 : Outport  PortName=Info  Element=ChlrPress
  Out Bus Element3 : Outport  PortName=Info  Element=CmpPwr
  Out Bus Element4 : Outport  PortName=Info  Element=Qcond
  wires:
  Switch6/1 -> Out Bus Element/1, [CoolTempOut]
  [ByPCmd] -> Switch6/2
  [CoolTempIn] -> Switch6/1
  ByPCmd/1 -> [ByPCmd]
  Divide/1 -> Minus/2
  [CoolTempIn] -> Minus/1
  CoolTempIn/1 -> Add/2, [CoolTempIn]
  CmpCmd/1 -> Transfer Fcn/1
  Transfer Fcn/1 -> Power Comp/1
  Subtract/1 -> 1-D Lookup Table/1
  [CoolTempIn] -> Subtract/2
  1-D Lookup Table/1 -> Power Evap/1
  Signal Specification/1 -> Unit Conversion/1
  Unit Conversion/1 -> Signal Specification1/1
  Gain1/1 -> Specific Heat/1
  Add/1 -> Gain1/1
  [CoolTempOut] -> Add/1
  Power Comp/1 -> Signal Specification/1
  Signal Specification1/1 -> [CmpPwr], Power Evap/2, Out Bus Element3/1
  Power Evap/1 -> Add1/2, Gain/1
  Gain/1 -> Divide/1
  Env/1 -> Bus Selector/1
  Bus Selector/1 -> Subtract/1  "<AmbTemp>"
  [CmpPwr] -> Add1/1
  Add1/1 -> Out Bus Element4/1
  Minus/1 -> Transfer Fcn1/1
  Transfer Fcn1/1 -> Switch6/3
  Product/1 -> No0Div/1
  Specific Heat/1 -> Product/1
  CoolMFlow/1 -> Product/2
  No0Div/1 -> Divide/2
  AirTempCondOut/1 -> Subtract1/1
  AirTempCondIn/1 -> Subtract1/2
  Subtract1/1 -> 1-D Lookup Table1/1
  1-D Lookup Table1/1 -> Out Bus Element1/1
  [CoolTempOut] -> Subtract3/2
  [CoolTempIn] -> Subtract3/1
  Subtract3/1 -> 1-D Lookup Table2/1
  1-D Lookup Table2/1 -> Out Bus Element2/1

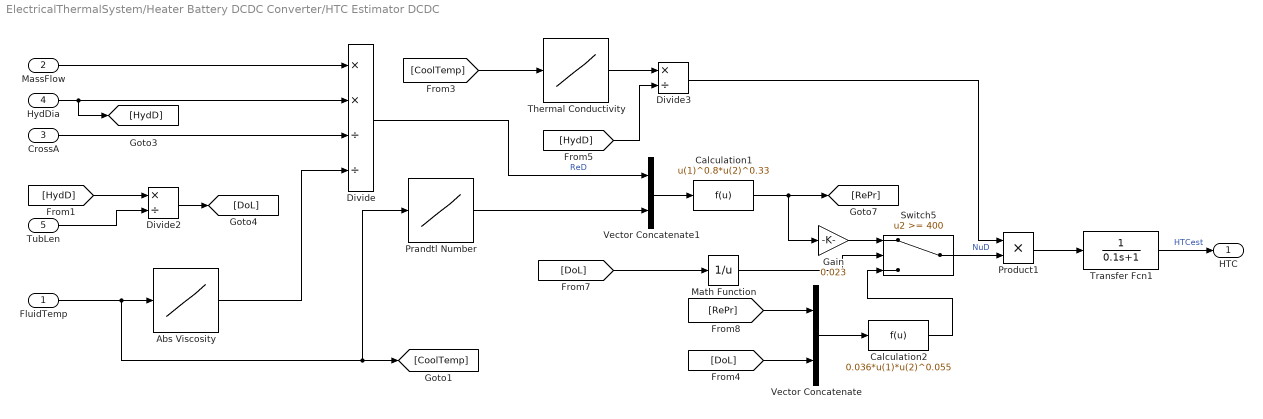
== system ElectricalThermalSystem/Heater Battery DCDC Converter/HTC Estimator DCDC ==
  FluidTemp : Inport
  MassFlow : Inport  Port=2
  CrossA : Inport  Port=3  OutMin=eps
  HydDia : Inport  Port=4
  TubLen : Inport  Port=5
  Abs Viscosity : Lookup_n-D  NumberOfTableDimensions=1  BreakpointsForDimension1=PlntThrCoolCpBpt  Table=PlntThrCoolVisc  ExtrapMethod=Clip  UseLastTableValue=on  InternalRulePriority=Speed  RndMeth=Simplest
  Calculation1 : Fcn  Expr=u(1)^0.8*u(2)^0.33
  Calculation2 : Fcn  Expr=0.036*u(1)*u(2)^0.055
  Divide : Product  Inputs=**//
  Divide2 : Product  Inputs=*/
  Divide3 : Product  Inputs=*/
  Gain : Gain  Gain=0.023
  Math Function : Math  Operator=reciprocal
  Prandtl Number : Lookup_n-D  NumberOfTableDimensions=1  BreakpointsForDimension1=PlntThrCoolCpBpt  Table=PlntThrCoolPrand  ExtrapMethod=Clip  UseLastTableValue=on  InternalRulePriority=Speed  RndMeth=Simplest
  Product1 : Product
  Switch5 : Switch  Threshold=400  SaturateOnIntegerOverflow=off  InputSameDT=off
  Thermal Conductivity : Lookup_n-D  NumberOfTableDimensions=1  BreakpointsForDimension1=PlntThrCoolCpBpt  Table=PlntThrCoolCond  ExtrapMethod=Clip  UseLastTableValue=on  InternalRulePriority=Speed  RndMeth=Simplest
  Transfer Fcn1 : TransferFcn  Denominator=[0.1 1]
  Vector Concatenate : Concatenate
  Vector Concatenate1 : Concatenate
  HTC : Outport
  wires:
  Transfer Fcn1/1 -> HTC/1  "HTCest"
  FluidTemp/1 -> Prandtl Number/1, [CoolTemp], Abs Viscosity/1
  [CoolTemp] -> Thermal Conductivity/1
  MassFlow/1 -> Divide/1
  HydDia/1 -> [HydD], Divide/2
  CrossA/1 -> Divide/3
  [HydD] -> Divide2/1
  TubLen/1 -> Divide2/2
  Divide2/1 -> [DoL]
  Abs Viscosity/1 -> Divide/4
  Divide/1 -> Vector Concatenate1/1  "ReD"
  Prandtl Number/1 -> Vector Concatenate1/2
  Vector Concatenate1/1 -> Calculation1/1
  [DoL] -> Math Function/1
  Math Function/1 -> Switch5/2
  Thermal Conductivity/1 -> Divide3/1
  [HydD] -> Divide3/2
  Divide3/1 -> Product1/1
  Gain/1 -> Switch5/1
  Calculation1/1 -> [RePr], Gain/1
  [RePr] -> Vector Concatenate/1
  [DoL] -> Vector Concatenate/2
  Vector Concatenate/1 -> Calculation2/1
  Calculation2/1 -> Switch5/3
  Switch5/1 -> Product1/2  "NuD"
  Product1/1 -> Transfer Fcn1/1

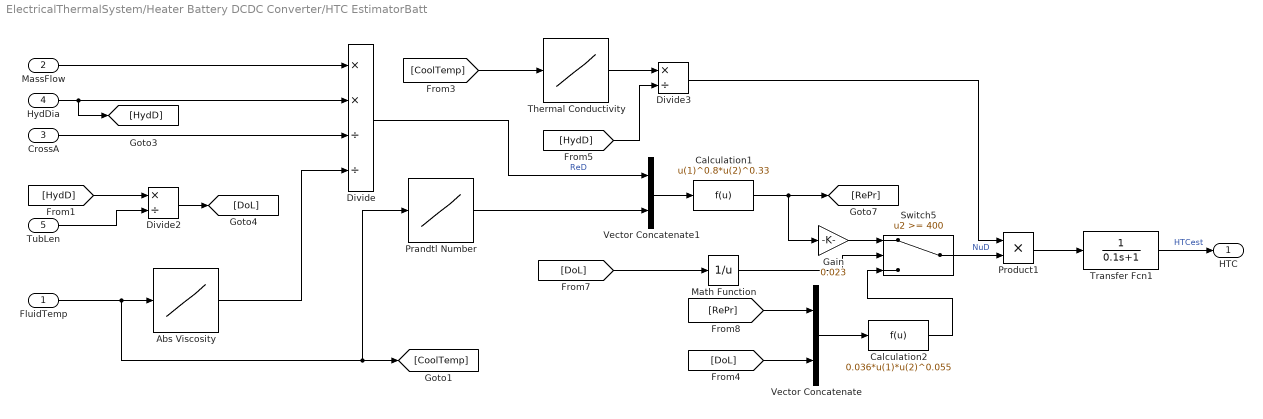
== system ElectricalThermalSystem/Heater Battery DCDC Converter/HTC EstimatorBatt ==
  FluidTemp : Inport
  MassFlow : Inport  Port=2
  CrossA : Inport  Port=3  OutMin=eps
  HydDia : Inport  Port=4
  TubLen : Inport  Port=5
  Abs Viscosity : Lookup_n-D  NumberOfTableDimensions=1  BreakpointsForDimension1=PlntThrCoolCpBpt  Table=PlntThrCoolVisc  ExtrapMethod=Clip  UseLastTableValue=on  InternalRulePriority=Speed  RndMeth=Simplest
  Calculation1 : Fcn  Expr=u(1)^0.8*u(2)^0.33
  Calculation2 : Fcn  Expr=0.036*u(1)*u(2)^0.055
  Divide : Product  Inputs=**//
  Divide2 : Product  Inputs=*/
  Divide3 : Product  Inputs=*/
  Gain : Gain  Gain=0.023
  Math Function : Math  Operator=reciprocal
  Prandtl Number : Lookup_n-D  NumberOfTableDimensions=1  BreakpointsForDimension1=PlntThrCoolCpBpt  Table=PlntThrCoolPrand  ExtrapMethod=Clip  UseLastTableValue=on  InternalRulePriority=Speed  RndMeth=Simplest
  Product1 : Product
  Switch5 : Switch  Threshold=400  SaturateOnIntegerOverflow=off  InputSameDT=off
  Thermal Conductivity : Lookup_n-D  NumberOfTableDimensions=1  BreakpointsForDimension1=PlntThrCoolCpBpt  Table=PlntThrCoolCond  ExtrapMethod=Clip  UseLastTableValue=on  InternalRulePriority=Speed  RndMeth=Simplest
  Transfer Fcn1 : TransferFcn  Denominator=[0.1 1]
  Vector Concatenate : Concatenate
  Vector Concatenate1 : Concatenate
  HTC : Outport
  wires:
  Transfer Fcn1/1 -> HTC/1  "HTCest"
  FluidTemp/1 -> Prandtl Number/1, [CoolTemp], Abs Viscosity/1
  [CoolTemp] -> Thermal Conductivity/1
  MassFlow/1 -> Divide/1
  HydDia/1 -> [HydD], Divide/2
  CrossA/1 -> Divide/3
  [HydD] -> Divide2/1
  TubLen/1 -> Divide2/2
  Divide2/1 -> [DoL]
  Abs Viscosity/1 -> Divide/4
  Divide/1 -> Vector Concatenate1/1  "ReD"
  Prandtl Number/1 -> Vector Concatenate1/2
  Vector Concatenate1/1 -> Calculation1/1
  [DoL] -> Math Function/1
  Math Function/1 -> Switch5/2
  Thermal Conductivity/1 -> Divide3/1
  [HydD] -> Divide3/2
  Divide3/1 -> Product1/1
  Gain/1 -> Switch5/1
  Calculation1/1 -> [RePr], Gain/1
  [RePr] -> Vector Concatenate/1
  [DoL] -> Vector Concatenate/2
  Vector Concatenate/1 -> Calculation2/1
  Calculation2/1 -> Switch5/3
  Switch5/1 -> Product1/2  "NuD"
  Product1/1 -> Transfer Fcn1/1

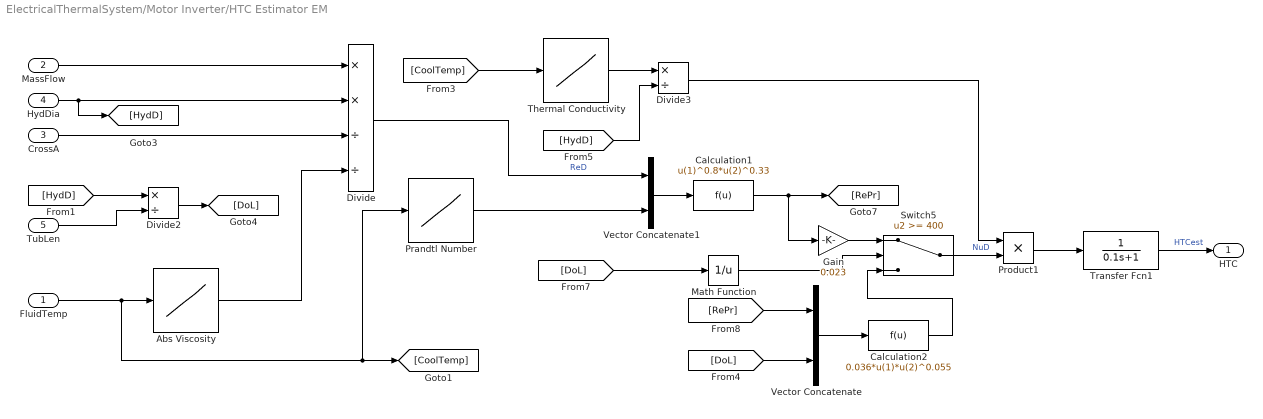
== system ElectricalThermalSystem/Motor Inverter/HTC Estimator EM ==
  FluidTemp : Inport
  MassFlow : Inport  Port=2
  CrossA : Inport  Port=3  OutMin=eps
  HydDia : Inport  Port=4
  TubLen : Inport  Port=5
  Abs Viscosity : Lookup_n-D  NumberOfTableDimensions=1  BreakpointsForDimension1=PlntThrCoolCpBpt  Table=PlntThrCoolVisc  ExtrapMethod=Clip  UseLastTableValue=on  InternalRulePriority=Speed  RndMeth=Simplest
  Calculation1 : Fcn  Expr=u(1)^0.8*u(2)^0.33
  Calculation2 : Fcn  Expr=0.036*u(1)*u(2)^0.055
  Divide : Product  Inputs=**//
  Divide2 : Product  Inputs=*/
  Divide3 : Product  Inputs=*/
  Gain : Gain  Gain=0.023
  Math Function : Math  Operator=reciprocal
  Prandtl Number : Lookup_n-D  NumberOfTableDimensions=1  BreakpointsForDimension1=PlntThrCoolCpBpt  Table=PlntThrCoolPrand  ExtrapMethod=Clip  UseLastTableValue=on  InternalRulePriority=Speed  RndMeth=Simplest
  Product1 : Product
  Switch5 : Switch  Threshold=400  SaturateOnIntegerOverflow=off  InputSameDT=off
  Thermal Conductivity : Lookup_n-D  NumberOfTableDimensions=1  BreakpointsForDimension1=PlntThrCoolCpBpt  Table=PlntThrCoolCond  ExtrapMethod=Clip  UseLastTableValue=on  InternalRulePriority=Speed  RndMeth=Simplest
  Transfer Fcn1 : TransferFcn  Denominator=[0.1 1]
  Vector Concatenate : Concatenate
  Vector Concatenate1 : Concatenate
  HTC : Outport
  wires:
  Transfer Fcn1/1 -> HTC/1  "HTCest"
  FluidTemp/1 -> Prandtl Number/1, [CoolTemp], Abs Viscosity/1
  [CoolTemp] -> Thermal Conductivity/1
  MassFlow/1 -> Divide/1
  HydDia/1 -> [HydD], Divide/2
  CrossA/1 -> Divide/3
  [HydD] -> Divide2/1
  TubLen/1 -> Divide2/2
  Divide2/1 -> [DoL]
  Abs Viscosity/1 -> Divide/4
  Divide/1 -> Vector Concatenate1/1  "ReD"
  Prandtl Number/1 -> Vector Concatenate1/2
  Vector Concatenate1/1 -> Calculation1/1
  [DoL] -> Math Function/1
  Math Function/1 -> Switch5/2
  Thermal Conductivity/1 -> Divide3/1
  [HydD] -> Divide3/2
  Divide3/1 -> Product1/1
  Gain/1 -> Switch5/1
  Calculation1/1 -> [RePr], Gain/1
  [RePr] -> Vector Concatenate/1
  [DoL] -> Vector Concatenate/2
  Vector Concatenate/1 -> Calculation2/1
  Calculation2/1 -> Switch5/3
  Switch5/1 -> Product1/2  "NuD"
  Product1/1 -> Transfer Fcn1/1

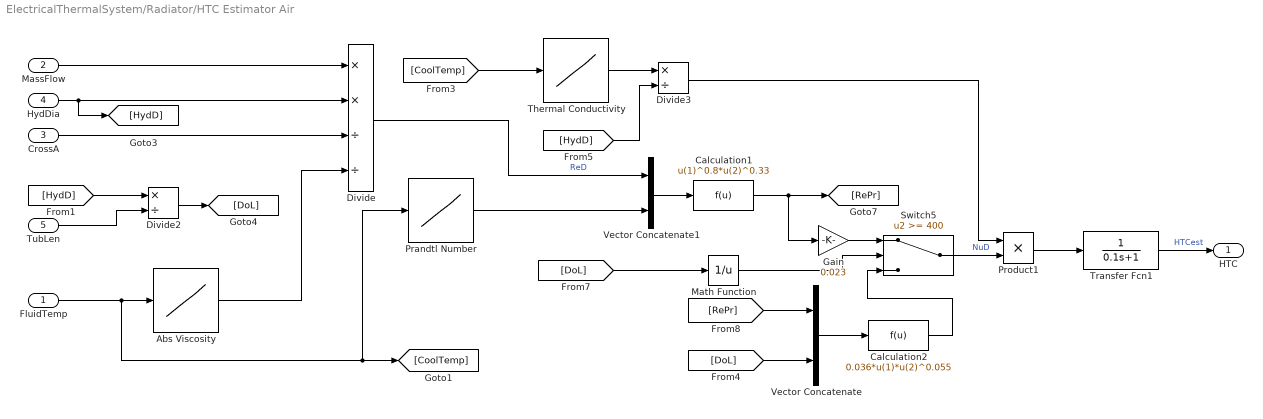
== system ElectricalThermalSystem/Radiator/HTC Estimator Air ==
  FluidTemp : Inport
  MassFlow : Inport  Port=2
  CrossA : Inport  Port=3  OutMin=eps
  HydDia : Inport  Port=4
  TubLen : Inport  Port=5
  Abs Viscosity : Lookup_n-D  NumberOfTableDimensions=1  BreakpointsForDimension1=PlntThrAirCpBpt  Table=PlntThrAirVisc  ExtrapMethod=Clip  UseLastTableValue=on  InternalRulePriority=Speed  RndMeth=Simplest
  Calculation1 : Fcn  Expr=u(1)^0.8*u(2)^0.33
  Calculation2 : Fcn  Expr=0.036*u(1)*u(2)^0.055
  Divide : Product  Inputs=**//
  Divide2 : Product  Inputs=*/
  Divide3 : Product  Inputs=*/
  Gain : Gain  Gain=0.023
  Math Function : Math  Operator=reciprocal
  Prandtl Number : Lookup_n-D  NumberOfTableDimensions=1  BreakpointsForDimension1=PlntThrAirCpBpt  Table=PlntThrAirPrand  ExtrapMethod=Clip  UseLastTableValue=on  InternalRulePriority=Speed  RndMeth=Simplest
  Product1 : Product
  Switch5 : Switch  Threshold=400  SaturateOnIntegerOverflow=off  InputSameDT=off
  Thermal Conductivity : Lookup_n-D  NumberOfTableDimensions=1  BreakpointsForDimension1=PlntThrAirCpBpt  Table=PlntThrAirCond  ExtrapMethod=Clip  UseLastTableValue=on  InternalRulePriority=Speed  RndMeth=Simplest
  Transfer Fcn1 : TransferFcn  Denominator=[0.1 1]
  Vector Concatenate : Concatenate
  Vector Concatenate1 : Concatenate
  HTC : Outport
  wires:
  Transfer Fcn1/1 -> HTC/1  "HTCest"
  FluidTemp/1 -> Prandtl Number/1, [CoolTemp], Abs Viscosity/1
  [CoolTemp] -> Thermal Conductivity/1
  MassFlow/1 -> Divide/1
  HydDia/1 -> [HydD], Divide/2
  CrossA/1 -> Divide/3
  [HydD] -> Divide2/1
  TubLen/1 -> Divide2/2
  Divide2/1 -> [DoL]
  Abs Viscosity/1 -> Divide/4
  Divide/1 -> Vector Concatenate1/1  "ReD"
  Prandtl Number/1 -> Vector Concatenate1/2
  Vector Concatenate1/1 -> Calculation1/1
  [DoL] -> Math Function/1
  Math Function/1 -> Switch5/2
  Thermal Conductivity/1 -> Divide3/1
  [HydD] -> Divide3/2
  Divide3/1 -> Product1/1
  Gain/1 -> Switch5/1
  Calculation1/1 -> [RePr], Gain/1
  [RePr] -> Vector Concatenate/1
  [DoL] -> Vector Concatenate/2
  Vector Concatenate/1 -> Calculation2/1
  Calculation2/1 -> Switch5/3
  Switch5/1 -> Product1/2  "NuD"
  Product1/1 -> Transfer Fcn1/1

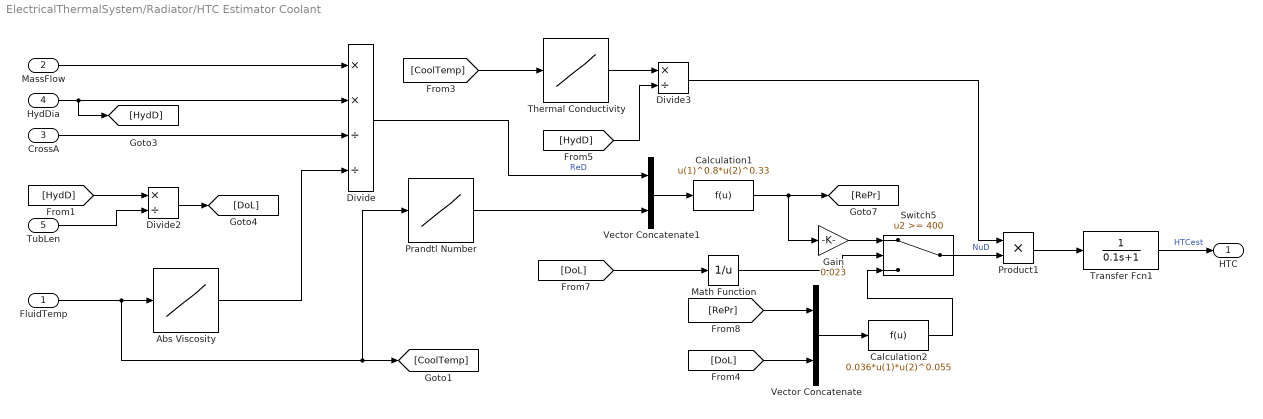
== system ElectricalThermalSystem/Radiator/HTC Estimator Coolant ==
  FluidTemp : Inport
  MassFlow : Inport  Port=2
  CrossA : Inport  Port=3  OutMin=eps
  HydDia : Inport  Port=4
  TubLen : Inport  Port=5
  Abs Viscosity : Lookup_n-D  NumberOfTableDimensions=1  BreakpointsForDimension1=PlntThrCoolCpBpt  Table=PlntThrCoolVisc  ExtrapMethod=Clip  UseLastTableValue=on  InternalRulePriority=Speed  RndMeth=Simplest
  Calculation1 : Fcn  Expr=u(1)^0.8*u(2)^0.33
  Calculation2 : Fcn  Expr=0.036*u(1)*u(2)^0.055
  Divide : Product  Inputs=**//
  Divide2 : Product  Inputs=*/
  Divide3 : Product  Inputs=*/
  Gain : Gain  Gain=0.023
  Math Function : Math  Operator=reciprocal
  Prandtl Number : Lookup_n-D  NumberOfTableDimensions=1  BreakpointsForDimension1=PlntThrCoolCpBpt  Table=PlntThrCoolPrand  ExtrapMethod=Clip  UseLastTableValue=on  InternalRulePriority=Speed  RndMeth=Simplest
  Product1 : Product
  Switch5 : Switch  Threshold=400  SaturateOnIntegerOverflow=off  InputSameDT=off
  Thermal Conductivity : Lookup_n-D  NumberOfTableDimensions=1  BreakpointsForDimension1=PlntThrCoolCpBpt  Table=PlntThrCoolCond  ExtrapMethod=Clip  UseLastTableValue=on  InternalRulePriority=Speed  RndMeth=Simplest
  Transfer Fcn1 : TransferFcn  Denominator=[0.1 1]
  Vector Concatenate : Concatenate
  Vector Concatenate1 : Concatenate
  HTC : Outport
  wires:
  Transfer Fcn1/1 -> HTC/1  "HTCest"
  FluidTemp/1 -> Prandtl Number/1, [CoolTemp], Abs Viscosity/1
  [CoolTemp] -> Thermal Conductivity/1
  MassFlow/1 -> Divide/1
  HydDia/1 -> [HydD], Divide/2
  CrossA/1 -> Divide/3
  [HydD] -> Divide2/1
  TubLen/1 -> Divide2/2
  Divide2/1 -> [DoL]
  Abs Viscosity/1 -> Divide/4
  Divide/1 -> Vector Concatenate1/1  "ReD"
  Prandtl Number/1 -> Vector Concatenate1/2
  Vector Concatenate1/1 -> Calculation1/1
  [DoL] -> Math Function/1
  Math Function/1 -> Switch5/2
  Thermal Conductivity/1 -> Divide3/1
  [HydD] -> Divide3/2
  Divide3/1 -> Product1/1
  Gain/1 -> Switch5/1
  Calculation1/1 -> [RePr], Gain/1
  [RePr] -> Vector Concatenate/1
  [DoL] -> Vector Concatenate/2
  Vector Concatenate/1 -> Calculation2/1
  Calculation2/1 -> Switch5/3
  Switch5/1 -> Product1/2  "NuD"
  Product1/1 -> Transfer Fcn1/1
